simulink model "vipcolorsegmentation"  (R2015b)
settings: Solver=FixedStepDiscrete  StartTime=0.0  StopTime=inf  RelTol=1e-3
PreLoadFcn:
  | max_num_blobs = 30;
  | % threshold to compare against distance
  | % between closest bounding box edges;
  | % if the distance in row and column direction
  | % is less than the specified threshold, bounding
  | % boxes are merged.
  | bbox_edge_distance_threshold = [3 3];
undefined symbols (not defined in the file or in its folder): gray, Rec, SDTV, strel
libraries: simulink x9, visionsinks x3, visionfilter x1, visionmorphops x1, visionanalysis x1, visionstatistics x1, visiontextngfix x1, vipmisc x1, visionconversions x1, dspvision x1
CloseFcn:
  | clear max_num_blobs;
  | clear bbox_edge_distance_threshold;
settings Model: FPTRunName=Active  ExtModeAutoUpdateStatusClock=off  Creator=The MathWorks, Inc.  LastModifiedBy=The MathWorks, Inc.
settings DataIOCC: SaveFormat=Array  SaveOutput=off  SignalLogging=off  SaveTime=off
settings OptimizationCC: ExpressionDepthLimit=2147483647  InitFltsAndDblsToZero=on  EfficientMapNaN2IntZero=off
settings DebuggingCC: SaveWithParameterizedLinksMsg=none  UnderspecifiedInitializationDetection=Classic  MergeDetectMultiDrivingBlocksExec=none  SignalResolutionControl=TryResolveAllWithWarning  SolverPrmCheckMsg=warning  MultiTaskDSMMsg=warning  MultiTaskCondExecSysMsg=none  SigSpecEnsureSampleTimeMsg=none  FcnCallInpInsideContextMsg=UseLocalSettings  StateNameClashWarn=warning  StrictBusMsg=None
settings HardwareCC: ProdBitPerPointer=32  ProdLargestAtomicFloat=None  ProdIntDivRoundTo=Undefined  ProdEndianess=Unspecified  ProdWordSize=32  ProdHWDeviceType=32-bit Generic  TargetBitPerLong=64  TargetBitPerPointer=64  TargetLongLongMode=on  TargetIntDivRoundTo=Zero  TargetEndianess=LittleEndian  TargetWordSize=64  TargetHWDeviceType=Generic->MATLAB Host Computer  ProdEqTarget=off
settings GRTTargetCC: TargetFcnLib=ansi_tfl_tmw.mat  GeneratePreprocessorConditionals=Disable all  CombineOutputUpdateFcns=off  GRTInterface=on
settings ConfigComp: CovModelRefEnable=Off

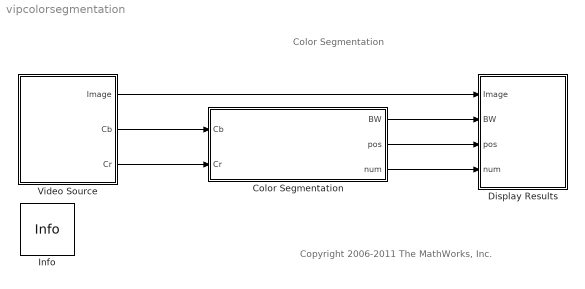
== system vipcolorsegmentation ==
  note: Color Segmentation
  note: Copyright 2006-2011 The MathWorks, Inc.
  Color Segmentation : Subsystem
  Display Results : Subsystem
  Info : vipmisc/Info  SystemSampleTime=-1
  "Video Source " : Subsystem
  wires:
  "Video Source "/2(Cb) -> Color Segmentation/1(Cb)
  "Video Source "/3(Cr) -> Color Segmentation/2(Cr)
  Color Segmentation/2(pos) -> Display Results/3(pos)
  Color Segmentation/3(num) -> Display Results/4(num)
  Color Segmentation/1(BW) -> Display Results/2(BW)
  "Video Source "/1(Image) -> Display Results/1(Image)

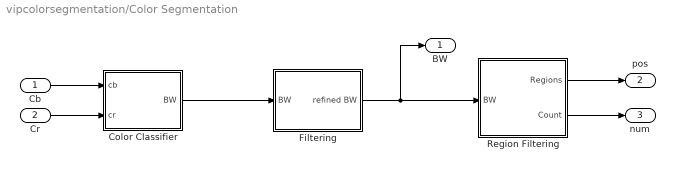
== system vipcolorsegmentation/Color Segmentation ==
  Cb : Inport
  Cr : Inport  Port=2
  Color Classifier : Subsystem
  Filtering : Subsystem
  Region Filtering : Subsystem
  BW : Outport
  pos : Outport  Port=2
  num : Outport  Port=3
  wires:
  Color Classifier/1(BW) -> Filtering/1(BW)
  Filtering/1(refined BW) -> BW/1, Region Filtering/1(BW)
  Cb/1 -> Color Classifier/1(cb)
  Cr/1 -> Color Classifier/2(cr)
  Region Filtering/1(Regions) -> pos/1
  Region Filtering/2(Count) -> num/1

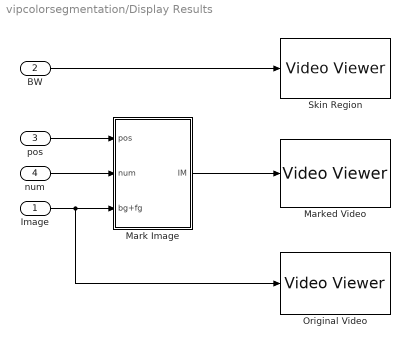
== system vipcolorsegmentation/Display Results ==
  Image : Inport
  BW : Inport  Port=2
  pos : Inport  Port=3
  num : Inport  Port=4
  Mark Image : Subsystem
  Marked Video : visionsinks/Video Viewer  inputType=Obsolete7b  imagePorts=One multidimensional signal  useColorMap=off  colormapValue=gray(256)  specRange=off  minInputVal=0  maxInputVal=255  FigPos=[410 344 166 142]  AxisZoom=on  trueSizedOnce=on  OpenAtMdlStart=on  DefaultConfigurationName=vipscopes.VideoViewerScopeCfg
  Original Video : visionsinks/Video Viewer  inputType=Obsolete7b  imagePorts=One multidimensional signal  useColorMap=off  colormapValue=gray(256)  specRange=off  minInputVal=0  maxInputVal=255  FigPos=[68 344 160 141]  AxisZoom=on  trueSizedOnce=on  OpenAtMdlStart=on  DefaultConfigurationName=vipscopes.VideoViewerScopeCfg
  Skin Region : visionsinks/Video Viewer  inputType=Obsolete7b  imagePorts=One multidimensional signal  useColorMap=off  colormapValue=gray(256)  specRange=off  minInputVal=0  maxInputVal=255  FigPos=[238 344 162 144]  AxisZoom=on  trueSizedOnce=on  OpenAtMdlStart=on  DefaultConfigurationName=vipscopes.VideoViewerScopeCfg
  wires:
  num/1 -> Mark Image/2(num)
  pos/1 -> Mark Image/1(pos)
  BW/1 -> Skin Region/1
  Mark Image/1(IM) -> Marked Video/1
  Image/1 -> Original Video/1, Mark Image/3(bg+fg)

== system vipcolorsegmentation/Video Source  ==
  Color Space Conversion : visionconversions/Color Space  Conversion  conversion=Obsolete  conversionActive=R'G'B' to Y'CbCr  wp_str=D65  rec=Rec. 601 (SDTV)  sys=1125/60/2:1  imagePorts=One multidimensional signal
  From Multimedia File : dspvision/From Multimedia File  inputFilename=vipcolorsegmentation.avi  loop=on  numPlays=inf  outputStreams=Video only  videoDataType=single  audioDataType=int16  inheritSampleTime=on  userDefinedSampleTime=1/30  noAudioOutput=off  isIntensityVideo=off  fourcc=RGB  colorVideoFormat=One multidimensional signal  outputEOF=off  dataOrg=Column-major  audioFrameSize=1024  computeAudioFrameSize=off  outSamplingMode=Frame based
  Select Cb : Selector  NumberOfDimensions=3  InputPortWidth=3  IndexOptions=Select all,Select all,Index vector (dialog)  Indices=[1 3],1,2  OutputSizes=1,1,1
  Select Cr : Selector  NumberOfDimensions=3  InputPortWidth=3  IndexOptions=Select all,Select all,Index vector (dialog)  Indices=[1 3],1,3  OutputSizes=1,1,1
  Image : Outport
  Cb : Outport  Port=2
  Cr : Outport  Port=3
  wires:
  From Multimedia File/1 -> Image/1, Color Space Conversion/1
  Color Space Conversion/1 -> Select Cb/1, Select Cr/1
  Select Cb/1 -> Cb/1
  Select Cr/1 -> Cr/1

== system vipcolorsegmentation/Color Segmentation/Color Classifier ==
  cb : Inport
  cr : Inport  Port=2
  2-D FIR Filter : visionfilter/2-D FIR Filter  separable=off  filtSrc=Specify via dialog  filterMtrx=single(1/9*ones(3))  verticalFilter=[4 0]  horizontalFilter=[4 0]  outSize=Full  padType=Constant  padSrc=Specify via dialog  padVal=0  method=Convolution  firstCoeffSignedness=Signed  firstCoeffDataTypeStr=Inherit: Same word length as input  firstCoeffLastDataTypeStr=Inherit: Same word length as input  firstCoeffMin=[]  firstCoeffMax=[]  outputMode=Binary point scaling  outputWordLength=32  outputFracLength=12  outputSignedness=Auto  outputDataTypeStr=fixdt([],32,12)  outputLastDataTypeStr=fixdt([],32,12)  outputMin=[]  outputMax=[]  accumDataTypeStr=Inherit: Same as product output  accumLastDataTypeStr=Inherit: Same as product output  prodOutputMode=Binary point scaling  prodOutputWordLength=32  prodOutputFracLength=10  prodOutputDataTypeStr=fixdt([],32,10)  prodOutputLastDataTypeStr=fixdt([],32,10)  roundingMode=Floor  overflowMode=off
  Compare To Constant1 : simulink/Logic and Bit Operations/Compare To Constant  relop=<  const=2.5  OutDataTypeStr=boolean  ZeroCross=off
  "Mahalanobis Distance " : Subsystem
  BW : Outport
  wires:
  "Mahalanobis Distance "/1(Distance) -> 2-D FIR Filter/1
  cb/1 -> "Mahalanobis Distance "/1(Cb)
  cr/1 -> "Mahalanobis Distance "/2(Cr)
  Compare To Constant1/1 -> BW/1
  2-D FIR Filter/1 -> Compare To Constant1/1

== system vipcolorsegmentation/Color Segmentation/Filtering ==
  BW : Inport
  Closing : visionmorphops/Closing  nhoodsrc=Specify via dialog  strel=strel('disk',5)
  Median Filter : Subsystem
  refined BW : Outport
  wires:
  BW/1 -> Median Filter/1(BW)
  Median Filter/1(Filtered BW) -> Closing/1
  Closing/1 -> refined BW/1

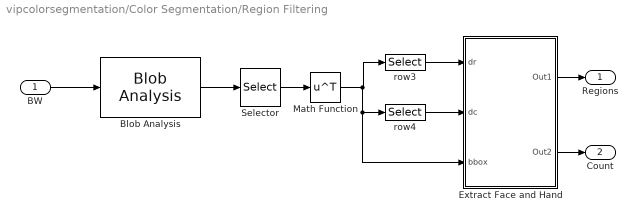
== system vipcolorsegmentation/Color Segmentation/Region Filtering ==
  BW : Inport
  Blob Analysis : visionstatistics/Blob Analysis  Tag=vipblks_row_conv  area=off  centroid=off  bBox=on  majorAxis=off  minorAxis=off  angle=off  eccentricity=off  equivDiameterSq=off  extent=off  perimeter=off  maxBlobs=max_num_blobs  warnIfNumBlobsExceeded=on  isCount=off  useMinArea=off  minArea=0  useMaxArea=off  maxArea=inf  excludeBorderBlob=off  outDT=single  isOutVarDim=on  isFill=on  fillValues=0  conn=8  isLabel=off  outputMode=Binary point scaling  outputWordLength=32  outputFracLength=16  firstCoeffMode=Binary point scaling  firstCoeffWordLength=16  firstCoeffFracLength=14  secondCoeffMode=Binary point scaling  secondCoeffWordLength=32  secondCoeffFracLength=16  accumMode=Binary point scaling  accumWordLength=32  accumFracLength=0  prodOutputMode=Binary point scaling  prodOutputWordLength=32  prodOutputFracLength=16  roundingMode=Floor  overflowMode=off
  Extract Face and Hand : Subsystem
  Math Function : Math  Operator=transpose  SaturateOnIntegerOverflow=on
  Selector : Selector  NumberOfDimensions=2  InputPortWidth=3  IndexOptions=Select all,Index vector (dialog)  Indices=[2 1 4 3],[2 1 4 3]  OutputSizes=1,1
  row3 : Selector  NumberOfDimensions=2  InputPortWidth=3  IndexOptions=Index vector (dialog),Select all  Indices=3,1  OutputSizes=1,1
  row4 : Selector  NumberOfDimensions=2  InputPortWidth=3  IndexOptions=Index vector (dialog),Select all  Indices=4,1  OutputSizes=1,1
  Regions : Outport
  Count : Outport  Port=2
  wires:
  row4/1 -> Extract Face and Hand/2(dc)
  row3/1 -> Extract Face and Hand/1(dr)
  Extract Face and Hand/2(Out2) -> Count/1
  Extract Face and Hand/1(Out1) -> Regions/1
  BW/1 -> Blob Analysis/1
  Selector/1 -> Math Function/1
  Blob Analysis/1 -> Selector/1
  Math Function/1 -> Extract Face and Hand/3(bbox), row4/1, row3/1

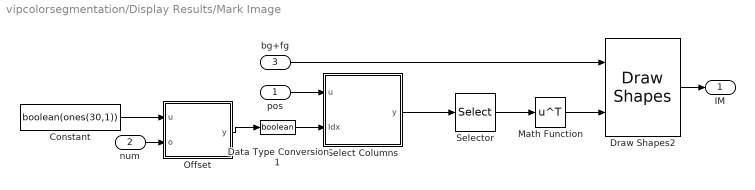
== system vipcolorsegmentation/Display Results/Mark Image ==
  pos : Inport
  num : Inport  Port=2
  bg+fg : Inport  Port=3
  Constant : Constant  Value=boolean(ones(30,1))
  Data Type Conversion1 : DataTypeConversion  OutDataTypeStr=boolean
  Draw Shapes2 : visiontextngfix/Draw Shapes  shape=Rectangles  fill=off  lineWidth=1  fillClrSource=Specify via dialog  display=User-specified value  intensity=200  color=[0 1 1]  opacity=0.6  viewport=Entire image  antialiasing=off  inType=Obsolete  imagePorts=One multidimensional signal  prodOutputMode=Binary point scaling  prodOutputWordLength=32  prodOutputFracLength=14  memoryMode=Specify word length  memoryWordLength=16  memoryFracLength=15  roundingMode=Floor  overflowMode=off
  Math Function : Math  Operator=transpose  SaturateOnIntegerOverflow=on
  Offset : MATLAB Function  TreatAsAtomicUnit=on
  Select Columns : MATLAB Function  TreatAsAtomicUnit=on
  Selector : Selector  NumberOfDimensions=2  InputPortWidth=3  IndexOptions=Index vector (dialog),Select all  Indices=[2 1 4 3],1  OutputSizes=1,1
  IM : Outport
  wires:
  Draw Shapes2/1 -> IM/1
  Data Type Conversion1/1 -> Select Columns/2(Idx)
  Constant/1 -> Offset/1(u)
  pos/1 -> Select Columns/1(u)
  num/1 -> Offset/2(o)
  bg+fg/1 -> Draw Shapes2/1
  Selector/1 -> Math Function/1
  Select Columns/1(y) -> Selector/1
  Math Function/1 -> Draw Shapes2/2
  Offset/1(y) -> Data Type Conversion1/1

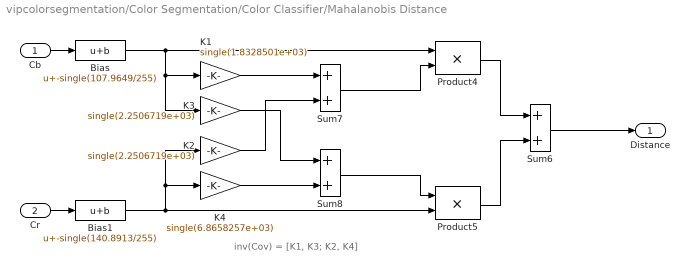
== system vipcolorsegmentation/Color Segmentation/Color Classifier/Mahalanobis Distance  ==
  note: inv(Cov) = [K1, K3; K2, K4]
  Cb : Inport
  Cr : Inport  Port=2
  Bias : Bias  Bias=-single(107.9649/255)
  Bias1 : Bias  Bias=-single(140.8913/255)
  K1 : Gain  Gain=single(1.8328501e+03)  SaturateOnIntegerOverflow=on  OutDataTypeStr=Inherit: Same as input  ParamDataTypeStr=Inherit: Same as input
  K2 : Gain  Gain=single(2.2506719e+03)  SaturateOnIntegerOverflow=on  OutDataTypeStr=Inherit: Same as input  ParamDataTypeStr=Inherit: Same as input
  K3 : Gain  Gain=single(2.2506719e+03)  SaturateOnIntegerOverflow=on  OutDataTypeStr=Inherit: Same as input  ParamDataTypeStr=Inherit: Same as input
  K4 : Gain  Gain=single(6.8658257e+03)  SaturateOnIntegerOverflow=on  OutDataTypeStr=Inherit: Same as input  ParamDataTypeStr=Inherit: Same as input
  Product4 : Product  SaturateOnIntegerOverflow=on  InputSameDT=on  OutDataTypeStr=Inherit: Same as first input
  Product5 : Product  SaturateOnIntegerOverflow=on  InputSameDT=on  OutDataTypeStr=Inherit: Same as first input
  Sum6 : Sum  SaturateOnIntegerOverflow=on  InputSameDT=on  OutDataTypeStr=Inherit: Same as first input
  Sum7 : Sum  SaturateOnIntegerOverflow=on  InputSameDT=on  OutDataTypeStr=Inherit: Same as first input
  Sum8 : Sum  SaturateOnIntegerOverflow=on  InputSameDT=on  OutDataTypeStr=Inherit: Same as first input
  Distance : Outport
  wires:
  Cb/1 -> Bias/1
  Cr/1 -> Bias1/1
  K4/1 -> Sum8/2
  Product4/1 -> Sum6/1
  Product5/1 -> Sum6/2
  K1/1 -> Sum7/1
  K2/1 -> Sum7/2
  K3/1 -> Sum8/1
  Sum7/1 -> Product4/2
  Sum8/1 -> Product5/1
  Bias/1 -> Product4/1, K1/1, K3/1
  Bias1/1 -> Product5/2, K4/1, K2/1
  Sum6/1 -> Distance/1

== system vipcolorsegmentation/Color Segmentation/Filtering/Median Filter ==
  BW : Inport
  Data Type Conversion5 : DataTypeConversion  OutDataTypeStr=boolean  SaturateOnIntegerOverflow=on  RndMeth=Zero
  Data Type Conversion6 : DataTypeConversion  OutDataTypeStr=single  SaturateOnIntegerOverflow=on  RndMeth=Zero
  Median Filter : visionanalysis/Median Filter  nghbood=[3 3]  outSize=Same as input port I  padType=Constant  padSrc=Specify via dialog  padVal=0  roundingMode=Floor  overflowMode=off
  Filtered BW : Outport
  wires:
  BW/1 -> Data Type Conversion6/1
  Data Type Conversion5/1 -> Filtered BW/1
  Median Filter/1 -> Data Type Conversion5/1
  Data Type Conversion6/1 -> Median Filter/1

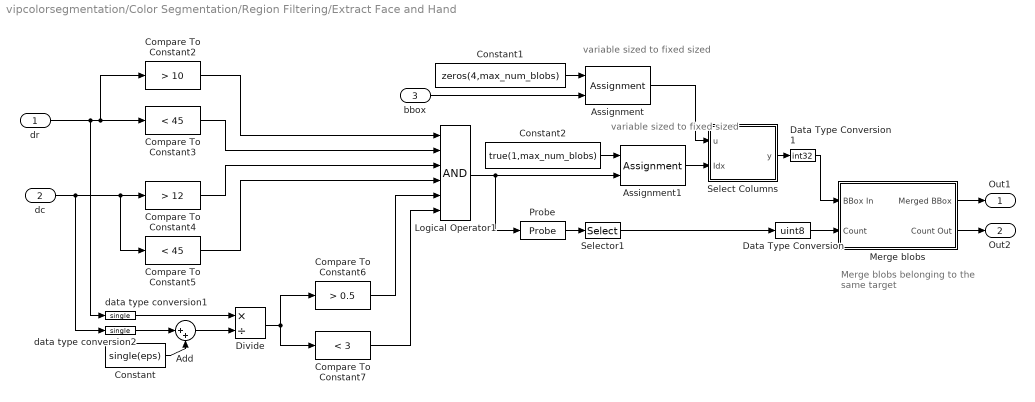
== system vipcolorsegmentation/Color Segmentation/Region Filtering/Extract Face and Hand ==
  note: Merge blobs belonging
      | to the same target
  note: variable sized to fixed sized
  note: variable sized to fixed sized
  dr : Inport
  dc : Inport  Port=2
  bbox : Inport  Port=3
  Add : Sum  Inputs=|++
  Assignment : Assignment  NumberOfDimensions=2  IndexMode=Zero-based  OutputInitialize=Specify size for each dimension in table  IndexOptions=Assign all,Starting index (dialog)  Indices=0,0  OutputSizes=1,1
  Assignment1 : Assignment  NumberOfDimensions=2  IndexMode=Zero-based  OutputInitialize=Specify size for each dimension in table  IndexOptions=Assign all,Starting index (dialog)  Indices=0,0  OutputSizes=1,1
  Compare To Constant2 : simulink/Logic and Bit Operations/Compare To Constant  relop=>  const=10  OutDataTypeStr=boolean  ZeroCross=off
  Compare To Constant3 : simulink/Logic and Bit Operations/Compare To Constant  relop=<  const=45  OutDataTypeStr=boolean  ZeroCross=off
  Compare To Constant4 : simulink/Logic and Bit Operations/Compare To Constant  relop=>  const=12  OutDataTypeStr=boolean  ZeroCross=off
  Compare To Constant5 : simulink/Logic and Bit Operations/Compare To Constant  relop=<  const=45  OutDataTypeStr=boolean  ZeroCross=off
  Compare To Constant6 : simulink/Logic and Bit Operations/Compare To Constant  relop=>  const=0.5  OutDataTypeStr=boolean  ZeroCross=off
  Compare To Constant7 : simulink/Logic and Bit Operations/Compare To Constant  relop=<  const=3  OutDataTypeStr=boolean  ZeroCross=off
  Constant : Constant  Value=single(eps)
  Constant1 : Constant  Value=zeros(4,max_num_blobs)  OutDataTypeStr=int32
  Constant2 : Constant  Value=true(1,max_num_blobs)  VectorParams1D=off
  Data Type Conversion : DataTypeConversion  OutDataTypeStr=uint8
  Data Type Conversion1 : DataTypeConversion  OutDataTypeStr=int32
  Divide : Product  Inputs=*/
  Logical Operator1 : Logic  Inputs=6  AllPortsSameDT=off  OutDataTypeStr=boolean
  Merge blobs : Subsystem
  Probe : Probe  ProbeWidth=off  ProbeSampleTime=off  ProbeComplexSignal=off  ProbeSignalDimensions=on  ProbeWidthDataType=uint8
  Select Columns : MATLAB Function  TreatAsAtomicUnit=on
  Selector1 : Selector  NumberOfDimensions=2  InputPortWidth=3  IndexOptions=Index vector (dialog),Index vector (dialog)  Indices=1,2  OutputSizes=99,1
  data type conversion1 : DataTypeConversion  OutDataTypeStr=single  SaturateOnIntegerOverflow=on  RndMeth=Zero
  data type conversion2 : DataTypeConversion  OutDataTypeStr=single  SaturateOnIntegerOverflow=on  RndMeth=Zero
  Out1 : Outport
  Out2 : Outport  Port=2
  wires:
  Merge blobs/1(Merged BBox) -> Out1/1
  data type conversion2/1 -> Add/1
  data type conversion1/1 -> Divide/1
  Compare To Constant7/1 -> Logical Operator1/6
  Compare To Constant6/1 -> Logical Operator1/5
  Divide/1 -> Compare To Constant7/1, Compare To Constant6/1
  Add/1 -> Divide/2
  dc/1 -> Compare To Constant4/1, Compare To Constant5/1, data type conversion2/1
  Compare To Constant5/1 -> Logical Operator1/4
  Compare To Constant4/1 -> Logical Operator1/3
  Compare To Constant3/1 -> Logical Operator1/2
  Compare To Constant2/1 -> Logical Operator1/1
  dr/1 -> Compare To Constant2/1, Compare To Constant3/1, data type conversion1/1
  Merge blobs/2(Count Out) -> Out2/1
  Data Type Conversion1/1 -> Merge blobs/1(BBox In)
  Constant/1 -> Add/2
  bbox/1 -> Assignment/2
  Constant1/1 -> Assignment/1
  Constant2/1 -> Assignment1/1
  Logical Operator1/1 -> Assignment1/2, Probe/1
  Assignment/1 -> Select Columns/1(u)
  Assignment1/1 -> Select Columns/2(Idx)
  Probe/1 -> Selector1/1
  Selector1/1 -> Data Type Conversion/1
  Data Type Conversion/1 -> Merge blobs/2(Count)
  Select Columns/1(y) -> Data Type Conversion1/1

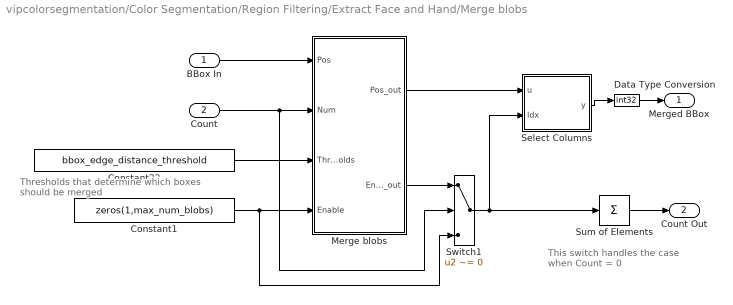
== system vipcolorsegmentation/Color Segmentation/Region Filtering/Extract Face and Hand/Merge blobs ==
  note: Thresholds that determine which boxes
      | should be merged
  note: This switch handles
      | the case when Count = 0
  BBox In : Inport
  Count : Inport  Port=2
  Constant1 : Constant  Value=zeros(1,max_num_blobs)  VectorParams1D=off  OutDataTypeStr=Inherit: Inherit via back propagation
  Constant22 : Constant  Value=bbox_edge_distance_threshold  VectorParams1D=off  OutDataTypeStr=Inherit: Inherit via back propagation
  Data Type Conversion : DataTypeConversion  OutDataTypeStr=int32
  Merge blobs : Subsystem
  Select Columns : MATLAB Function  TreatAsAtomicUnit=on
  Sum of Elements : Sum  Inputs=+
  Switch1 : Switch  Criteria=u2 ~= 0  Threshold=1  ZeroCross=off
  Merged BBox : Outport
  Count Out : Outport  Port=2
  wires:
  Constant22/1 -> Merge blobs/3(Thresholds)
  BBox In/1 -> Merge blobs/1(Pos)
  Data Type Conversion/1 -> Merged BBox/1
  Switch1/1 -> Sum of Elements/1, Select Columns/2(Idx)
  Merge blobs/2(Enable_out) -> Switch1/1
  Merge blobs/1(Pos_out) -> Select Columns/1(u)
  Constant1/1 -> Merge blobs/4(Enable), Switch1/3
  Count/1 -> Merge blobs/2(Num), Switch1/2
  Sum of Elements/1 -> Count Out/1
  Select Columns/1(y) -> Data Type Conversion/1

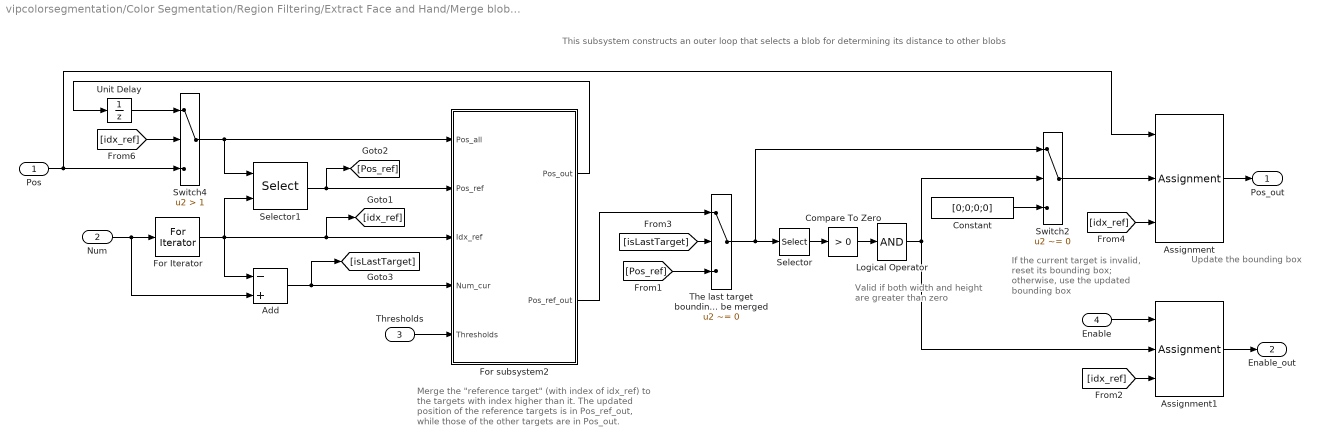
== system vipcolorsegmentation/Color Segmentation/Region Filtering/Extract Face and Hand/Merge blobs/Merge blobs ==
  note: Merge the "reference target" (with index of idx_ref)
      | to the targets with index higher than it.
      | The updated position of the reference targets
      | is in Pos_ref_out, while those of
      | the other targets are in Pos_out.
  note: This subsystem constructs an outer loop that selects a blob for determining its distance to other blobs
  note: Update the bounding box
  note: If the current target is invalid,
      | reset its bounding box;
      | otherwise, use the
      | updated bounding box
  note: Valid if both width and height
      | are greater than zero
  Pos : Inport
  Num : Inport  Port=2
  Thresholds : Inport  Port=3
  Enable : Inport  Port=4
  Add : Sum  Inputs=-+
  Assignment : Assignment  NumberOfDimensions=2  IndexOptions=Assign all,Index vector (port)  Indices=(-1),(-1)  OutputSizes=1, 1
  Assignment1 : Assignment  NumberOfDimensions=2  IndexOptions=Assign all,Index vector (port)  Indices=(-1),(-1)  OutputSizes=1, 1
  Compare To Zero : simulink/Logic and Bit Operations/Compare To Zero  relop=>  OutDataTypeStr=boolean  ZeroCross=off
  Constant : Constant  Value=[0;0;0;0]  OutDataTypeStr=Inherit: Inherit via back propagation
  For Iterator : ForIterator  ResetStates=reset  IterationSource=external
  For subsystem2 : Subsystem
  Logical Operator : Logic  Inputs=1  AllPortsSameDT=off  OutDataTypeStr=boolean
  Selector : Selector  InputPortWidth=4  IndexOptions=Index vector (dialog)  Indices=([3 4])  OutputSizes=1
  Selector1 : Selector  NumberOfDimensions=2  InputPortWidth=3  IndexOptions=Select all,Index vector (port)  Indices=(-1),(-1)  OutputSizes=1
  Switch2 : Switch  Criteria=u2 ~= 0  Threshold=1
  Switch4 : Switch  Criteria=u2 > Threshold  Threshold=1  InputSameDT=on
  The last target bounding box does not need to be merged : Switch  Criteria=u2 ~= 0  Threshold=1
  Unit Delay : UnitDelay  SampleTime=-1
  Pos_out : Outport
  Enable_out : Outport  Port=2
  wires:
  Enable/1 -> Assignment1/1
  Num/1 -> For Iterator/1, Add/2
  Switch4/1 -> For subsystem2/1(Pos_all), Selector1/1
  Selector1/1 -> For subsystem2/2(Pos_ref), [Pos_ref]
  Assignment1/1 -> Enable_out/1
  Selector/1 -> Compare To Zero/1
  Compare To Zero/1 -> Logical Operator/1
  Thresholds/1 -> For subsystem2/5(Thresholds)
  Unit Delay/1 -> Switch4/1
  Pos/1 -> Switch4/3, Assignment/1
  Logical Operator/1 -> Assignment1/2, Switch2/2
  Constant/1 -> Switch2/3
  Assignment/1 -> Pos_out/1
  [idx_ref] -> Assignment1/3
  For Iterator/1 -> Selector1/2, For subsystem2/3(Idx_ref), [idx_ref], Add/1
  Add/1 -> For subsystem2/4(Num_cur), [isLastTarget]
  [idx_ref] -> Assignment/3
  [idx_ref] -> Switch4/2
  For subsystem2/1(Pos_out) -> Unit Delay/1
  The last target bounding box does not need to be merged/1 -> Switch2/1, Selector/1
  Switch2/1 -> Assignment/2
  For subsystem2/2(Pos_ref_out) -> The last target bounding box does not need to be merged/1
  [isLastTarget] -> The last target bounding box does not need to be merged/2
  [Pos_ref] -> The last target bounding box does not need to be merged/3

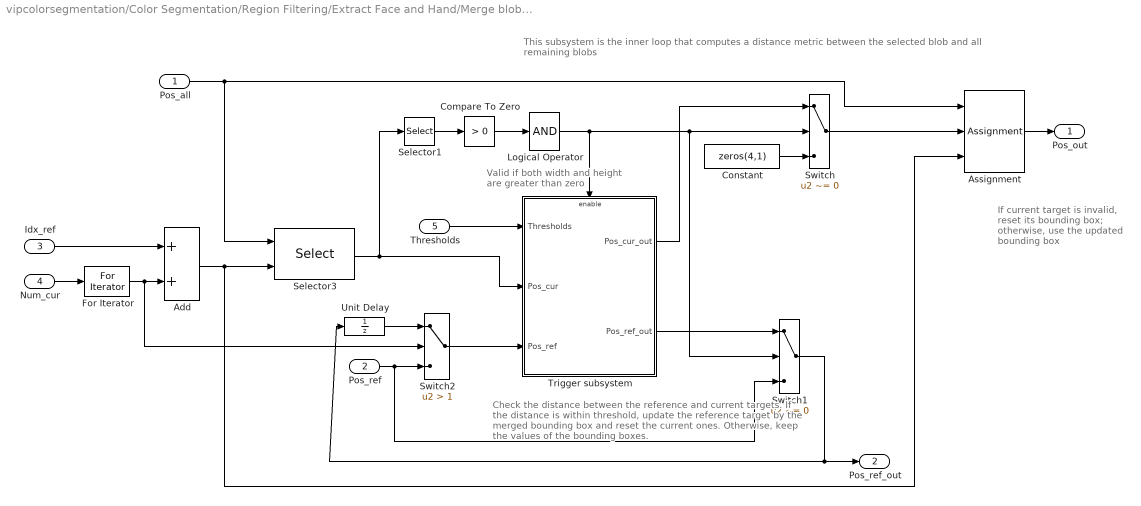
== system vipcolorsegmentation/Color Segmentation/Region Filtering/Extract Face and Hand/Merge blobs/Merge blobs/For subsystem2 ==
  note: Check the distance between the reference and current targets.
      | If the distance is within threshold, update the reference target
      | by the merged bounding box and reset the current ones.
      | Otherwise, keep the values of the bounding boxes.
  note: This subsystem is the inner loop that computes a distance metric between the selected blob and all remaining blobs
  note: If current target is invalid,
      | reset its bounding box;
      | otherwise, use the
      | updated bounding box
  note: Valid if both width and height
      | are greater than zero
  Pos_all : Inport
  Pos_ref : Inport  Port=2
  Idx_ref : Inport  Port=3
  Num_cur : Inport  Port=4
  Thresholds : Inport  Port=5
  Add : Sum
  Assignment : Assignment  NumberOfDimensions=2  IndexOptions=Assign all,Index vector (port)  Indices=(-1),(-1)  OutputSizes=1, 1
  Compare To Zero : simulink/Logic and Bit Operations/Compare To Zero  relop=>  OutDataTypeStr=boolean  ZeroCross=off
  Constant : Constant  Value=zeros(4,1)  VectorParams1D=off  OutDataTypeStr=Inherit: Inherit via back propagation
  For Iterator : ForIterator  ResetStates=reset  IterationSource=external
  Logical Operator : Logic  Inputs=1  AllPortsSameDT=off  OutDataTypeStr=boolean
  Selector1 : Selector  InputPortWidth=4  IndexOptions=Index vector (dialog)  Indices=([3 4])  OutputSizes=1
  Selector3 : Selector  NumberOfDimensions=2  InputPortWidth=3  IndexOptions=Select all,Index vector (port)  Indices=(-1),(-1)  OutputSizes=1
  Switch : Switch  Criteria=u2 ~= 0
  Switch1 : Switch  Criteria=u2 ~= 0
  Switch2 : Switch  Criteria=u2 > Threshold  Threshold=1
  Trigger subsystem : Subsystem
  Unit Delay : UnitDelay  SampleTime=-1
  Pos_out : Outport
  Pos_ref_out : Outport  Port=2
  wires:
  Pos_ref/1 -> Switch2/3, Switch1/3
  Unit Delay/1 -> Switch2/1
  Constant/1 -> Switch/3
  Trigger subsystem/1(Pos_cur_out) -> Switch/1
  Switch/1 -> Assignment/2
  Switch2/1 -> Trigger subsystem/3(Pos_ref)
  Logical Operator/1 -> Trigger subsystem/Enable, Switch/2, Switch1/2
  Compare To Zero/1 -> Logical Operator/1
  Selector1/1 -> Compare To Zero/1
  Selector3/1 -> Selector1/1, Trigger subsystem/2(Pos_cur)
  Assignment/1 -> Pos_out/1
  Thresholds/1 -> Trigger subsystem/1(Thresholds)
  Add/1 -> Selector3/2, Assignment/3
  Pos_all/1 -> Selector3/1, Assignment/1
  Num_cur/1 -> For Iterator/1
  For Iterator/1 -> Add/2, Switch2/2
  Idx_ref/1 -> Add/1
  Trigger subsystem/2(Pos_ref_out) -> Switch1/1
  Switch1/1 -> Pos_ref_out/1, Unit Delay/1

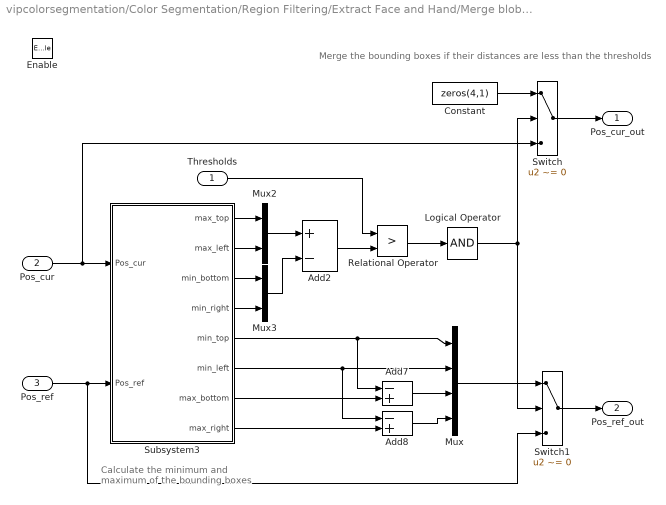
== system vipcolorsegmentation/Color Segmentation/Region Filtering/Extract Face and Hand/Merge blobs/Merge blobs/For subsystem2/Trigger subsystem ==
  note: Calculate the minimum and
      | maximum of the bounding boxes
  note: Merge the bounding boxes if their distances are less than the thresholds
  Thresholds : Inport
  Pos_cur : Inport  Port=2
  Pos_ref : Inport  Port=3
  Enable : EnablePort  PropagateVarSize=During execution
  Add2 : Sum  Inputs=+-
  Add7 : Sum  Inputs=-+
  Add8 : Sum  Inputs=-+
  Constant : Constant  Value=zeros(4,1)  VectorParams1D=off  OutDataTypeStr=Inherit: Inherit via back propagation
  Logical Operator : Logic  Inputs=1  AllPortsSameDT=off  OutDataTypeStr=boolean
  Mux : Mux
  Mux2 : Mux  Inputs=2
  Mux3 : Mux  Inputs=2
  Relational Operator : RelationalOperator  Operator=>  OutDataTypeStr=boolean
  Subsystem3 : Subsystem
  Switch : Switch  Criteria=u2 ~= 0
  Switch1 : Switch  Criteria=u2 ~= 0
  Pos_cur_out : Outport
  Pos_ref_out : Outport  Port=2
  wires:
  Add2/1 -> Relational Operator/2
  Mux3/1 -> Add2/2
  Mux2/1 -> Add2/1
  Subsystem3/3(min_bottom) -> Mux3/1
  Subsystem3/4(min_right) -> Mux3/2
  Subsystem3/2(max_left) -> Mux2/2
  Subsystem3/1(max_top) -> Mux2/1
  Logical Operator/1 -> Switch/2, Switch1/2
  Pos_cur/1 -> Switch/3, Subsystem3/1(Pos_cur)
  Switch/1 -> Pos_cur_out/1
  Switch1/1 -> Pos_ref_out/1
  Constant/1 -> Switch/1
  Mux/1 -> Switch1/1
  Add8/1 -> Mux/4
  Add7/1 -> Mux/3
  Subsystem3/8(max_right) -> Add8/2
  Subsystem3/6(min_left) -> Add8/1, Mux/2
  Subsystem3/7(max_bottom) -> Add7/2
  Subsystem3/5(min_top) -> Add7/1, Mux/1
  Pos_ref/1 -> Subsystem3/2(Pos_ref), Switch1/3
  Thresholds/1 -> Relational Operator/1
  Relational Operator/1 -> Logical Operator/1

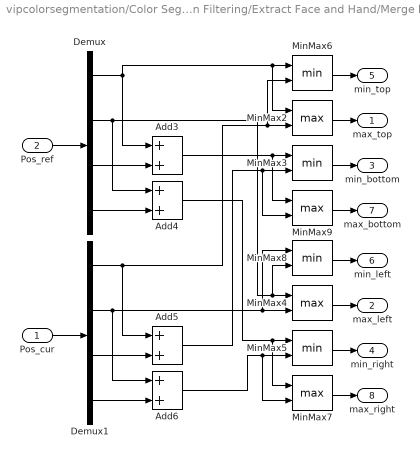
== system vipcolorsegmentation/Color Segmentation/Region Filtering/Extract Face and Hand/Merge blobs/Merge blobs/For subsystem2/Trigger subsystem/Subsystem3 ==
  Pos_cur : Inport
  Pos_ref : Inport  Port=2
  Add{3..6} (4 alike) : Sum
  Demux : Demux
  Demux1 : Demux
  MinMax{2,4,7,9} (4 alike) : MinMax  Function=max  Inputs=2
  MinMax{3,5..6,8} (4 alike) : MinMax  Inputs=2
  max_top : Outport
  max_left : Outport  Port=2
  min_bottom : Outport  Port=3
  min_right : Outport  Port=4
  min_top : Outport  Port=5
  min_left : Outport  Port=6
  max_bottom : Outport  Port=7
  max_right : Outport  Port=8
  wires:
  MinMax7/1 -> max_right/1
  MinMax5/1 -> min_right/1
  MinMax4/1 -> max_left/1
  MinMax8/1 -> min_left/1
  MinMax9/1 -> max_bottom/1
  MinMax3/1 -> min_bottom/1
  MinMax2/1 -> max_top/1
  MinMax6/1 -> min_top/1
  Pos_cur/1 -> Demux1/1
  Pos_ref/1 -> Demux/1
  Demux/2 -> MinMax8/2, MinMax4/1, Add4/1
  Demux/3 -> Add3/2
  Demux/4 -> Add4/2
  Demux1/2 -> MinMax8/1, MinMax4/2, Add6/1
  Demux1/3 -> Add5/2
  Demux1/4 -> Add6/2
  Demux/1 -> MinMax2/1, MinMax6/1, Add3/1
  Demux1/1 -> MinMax6/2, MinMax2/2, Add5/1
  Add3/1 -> MinMax9/1, MinMax3/1
  Add5/1 -> MinMax9/2, MinMax3/2
  Add4/1 -> MinMax7/1, MinMax5/1
  Add6/1 -> MinMax7/2, MinMax5/2

== matlab function vipcolorsegmentation/Display Results/Mark Image/Select Columns ==
  data: u input; y output; Idx input
function y = fcn(u, Idx)
%#codegen

y=zeros(size(u));
y(:,1:length(find(Idx))) = u(:,Idx);

== matlab function vipcolorsegmentation/Color Segmentation/Region Filtering/Extract Face and Hand/Select Columns ==
  data: u input; y output; Idx input
function y = fcn(u, Idx)
%#codegen

y=zeros(size(u));
y(:,1:length(find(Idx))) = u(:,Idx);

== matlab function vipcolorsegmentation/Display Results/Mark Image/Offset ==
  data: u input; y output; o input
function y = fcn(u, o)
%#codegen

y=zeros(size(u));
y(1:o) = u(1:o);

== matlab function vipcolorsegmentation/Color Segmentation/Region Filtering/Extract Face and Hand/Merge blobs/Select Columns ==
  data: u input; y output; Idx input
function y = fcn(u, Idx)
%#codegen

y=zeros(size(u));
y(:,:)=-1;
y(:,1:length(find(Idx))) = u(:,Idx);
